simulink model "lti_simulink2"  (Simulink 4.00)
settings: Solver=ode45  StartTime=0.0  StopTime=10.0  RelTol=1e-3
libraries: cstblocks x3, simulink3 x1
settings Model: LastModifiedBy=Administrator  Refine=3  BlockReductionOpt=off

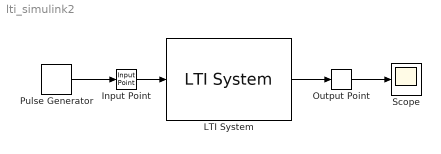
== system lti_simulink2 ==
  Input Point : cstblocks/Input Point
  LTI System : cstblocks/LTI System  sys=tf(1,[0.002 0.02 1])  IC=0
  Output Point : cstblocks/Output Point
  Pulse Generator : simulink3/Sources/Pulse Generator  period=4  duty=50  amplitude=1  start=0
  Scope : Scope
      settings: TimeRange=auto  YMin=-5  YMax=5  SaveToWorkspace=off  SaveName=ScopeData  LimitDataPoints=on  MaxDataPoints=5000
  wires:
  Pulse Generator/1 -> Input Point/1
  LTI System/1 -> Output Point/1
  Input Point/1 -> LTI System/1
  Output Point/1 -> Scope/1
